simulink model "untitled"  (Simulink 7.1)
settings: Solver=ode45  StartTime=0.0  StopTime=29.9  RelTol=1e-3
undefined symbols (not defined in the file): sfunyst
settings Model: Creator=Slavi  LastModifiedBy=Slavi

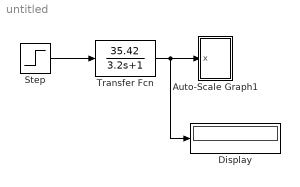
== system untitled ==
  Auto-Scale Graph1 : Subsystem  mask(Storage scope.){@1=2, @2=-10, @3=10, @4=200000, @5='b-/g--/c-./w:/m*/ro/b+'}
      mask prompts: @1 "Initial Time Range:"; @2 "Initial y-min:"; @3 "Initial y-max:"; @4 "Storage pts.:"; @5 "Line type (rgbw-.:xo):"
      mask help:
      | Storage scope using MATLAB graph window.
      | Enter plotting ranges and line type.
      mask init:
      | npts = @4; color = @5; ax = [0, @1, @2, @3]; dt=-1;
      mask Help: This block uses a MATLAB figure window to plot the input signal.  The graph limits are automatically scaled to the min and max values of the signal stored in the scope's signal buffer.  Line type must be in quotes.  See the M-file sfunyst.m.
      mask Display: plot(0,0,100,100,[83,76,63,52,42,38,28,16,11,84,11,11,11,90,90,11],[75,58,47,54,72,80,84,74,65,65,65,90,40,40,90,90])
  Display : Display
  Step : Step  Time=0  After=0.48  SampleTime=0
  Transfer Fcn : TransferFcn  Numerator=[35.42]  Denominator=[3.2 1]
  wires:
  Transfer Fcn/1 -> Auto-Scale Graph1/1(x), Display/1
  Step/1 -> Transfer Fcn/1

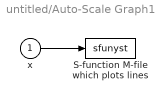
== system untitled/Auto-Scale Graph1 ==
  x : Inport
  "S-function M-file which plots lines " : S-Function  LoadFcn=sfunyst([],[],[],'LoadBlock')  FunctionName=sfunyst  Parameters=ax, color, npts, dt  EnableBusSupport=off
      settings: CopyFcn=sfunyst([],[],[],'CopyBlock')  DeleteFcn=sfunyst([],[],[],'DeleteBlock')
  wires:
  x/1 -> "S-function M-file which plots lines "/1
